simulink library "HybridFEMLibrary"  (Simulink 7.0)
values from neighbouring files (symbols this model uses):
  SampleRate = Integrator.Timestep    [HybridFEMSetupExample.m]
undefined symbols (not defined in the file or in its folder): Elements
libraries: simulink x2
settings Model: Creator=Tommy  LastModifiedBy=Tommy

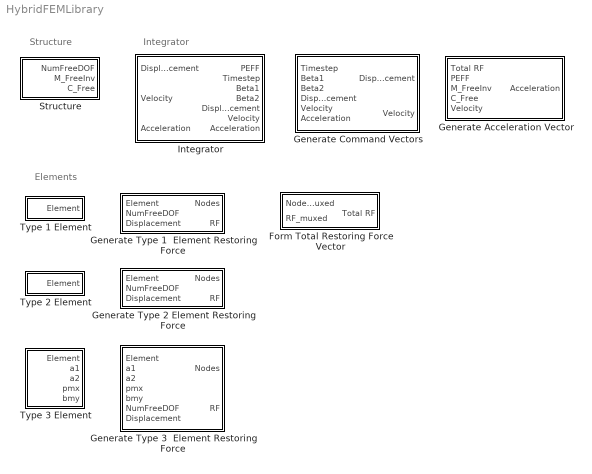
== system HybridFEMLibrary ==
  note: Elements
  note: Structure
  note: Integrator
  Form Total Restoring Force Vector : Subsystem
      mask Type: Form Restoring Force Vector
      mask Description:
      | Takes the restoring force vectors from each Element and combines them to form a total restoring force vector.
      | 
      | Connect the "Nodes_muxed" signal to the output of a Mux block which takes in all the Element "Nodes" outputs in order of ID.
      | 
      | Connect the "RF_muxed" signal to the output of a Mux block which takes in all the Element "RF" outputs in order of ID.
  Generate Acceleration Vector : Subsystem
      mask Type: Generate Acceleration Vector
      mask Description:
      | Takes the total restoring force vector and Integration parameters and generates the next step acceleration vector.
      | 
      | Connect the "Total RF" input to the output of the "Form Total Restoring Force Vector" block.
      | 
      | Connect the "PEFF", "M_Free_Inv" (MassMatrixFreeInv) and "C_Free" (DampingMatrixFree) to the "Structure" block.
      | 
      | Connect the "Velocity" input to the output of the "Generate Command Vectors" block
  Generate Command Vectors : Subsystem
      mask Type: Generate Command Vectors
      mask Description:
      | Generates the Displacement and Velocity vectors using the CR Algorithm.
      | 
      | Connect all inputs to the outputs of the "Integrator" block.
  Generate Type 1  Element Restoring Force : Subsystem
      mask Type: Generate Type 1 Element Restoring Force
      mask Description:
      | Generates the Restoring Force vector for a Type 1 Element
      | 
      | Connect the "Element" input to a "Type 1 Element" block.
      | 
      | Connect the "NumFreeDOF" input to the output of a "Structure" block.
      | 
      | Connect the "Displacement" input to the output of the "Generate Command Vectors" block.
  Generate Type 2 Element Restoring Force : Subsystem
      mask Type: Generate Type 2 Element Restoring Force
      mask Description:
      | Generates the Restoring Force vector for a Type 2 Element
      | 
      | Connect the "Element" input to a "Type 2 Element" block.
      | 
      | Connect the "NumFreeDOF" input to the output of a "Structure" block.
      | 
      | Connect the "Displacement" input to the output of the "Generate Command Vectors" block.
  Generate Type 3  Element Restoring Force : Subsystem
      mask Type: Generate Type 3 Element Restoring Force
      mask Description:
      | Generates the Restoring Force vector for a Type 3 Element
      | 
      | Connect the "Element" input to a "Type 3 Element" block.
      | 
      | Connect the "a1", "a2", "pmx" and "bmy" inputs to the outputs of the "Type 3 Element" block.
      | 
      | Connect the "NumFreeDOF" input to the output of a "Structure" block.
      | 
      | Connect the "Displacement" input to the output of the "Generate Command Vectors" block.
  Integrator : Subsystem
      mask Type: Integrator
      mask Description:
      | The Integrator structure is pulled from the MATLAB workspace after running the initialization script.
      | 
      | Connect the Displacement and Velocity inputs to the outputs of the "Generate Command Vectors" block.
      | 
      | Connect the Acceleration input to the output of the "Generate Acceleration Vector" block
  Structure : Subsystem
      mask Type: Structure Data Source
      mask Description: The Structure data is pulled from the MATLAB workspace after running the initialization file
  "Type 1 Element " : Subsystem  mask(Element Type 1){id=1}
      mask prompts: id "Element ID:"
      mask help: Enter the ID for this element corresponding with the input configuration file
  Type 2 Element : Subsystem  mask(Element Type 2){id=7}
      mask prompts: id "Element ID:"
      mask help: Enter the ID for this element corresponding with the input configuration file
  "Type 3 Element " : Subsystem  mask(Element Type 3){id=0}
      mask prompts: id "Element ID:"
      mask help: Enter the ID for this element corresponding with the input configuration file

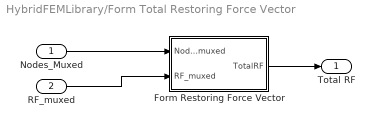
== system HybridFEMLibrary/Form Total Restoring Force Vector ==
  Nodes_Muxed : Inport  OutDataType=sfix(16)  OutScaling=2^0
  RF_muxed : Inport  Port=2  OutDataType=sfix(16)  OutScaling=2^0
  Form Restoring Force Vector : Stateflow chart
  Total RF : Outport  OutDataType=sfix(16)  OutScaling=2^0
  wires:
  Nodes_Muxed/1 -> Form Restoring Force Vector/1(Nodes_muxed)
  Form Restoring Force Vector/1(TotalRF) -> Total RF/1
  RF_muxed/1 -> Form Restoring Force Vector/2(RF_muxed)

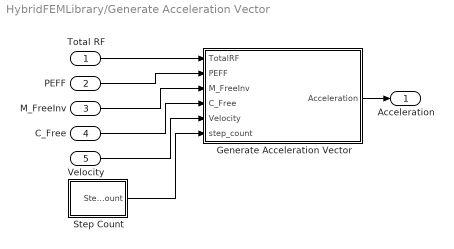
== system HybridFEMLibrary/Generate Acceleration Vector ==
  Total RF : Inport  OutDataType=sfix(16)  OutScaling=2^0
  PEFF : Inport  Port=2  OutDataType=sfix(16)  OutScaling=2^0
  M_FreeInv : Inport  Port=3  OutDataType=sfix(16)  OutScaling=2^0
  C_Free : Inport  Port=4  OutDataType=sfix(16)  OutScaling=2^0
  Velocity : Inport  Port=5  OutDataType=sfix(16)  OutScaling=2^0
  Generate Acceleration Vector : Stateflow chart
  Step Count : Subsystem
      mask Type: Step count
      mask Description: Generates the step count
  Acceleration : Outport  OutDataType=sfix(16)  OutScaling=2^0
  wires:
  Velocity/1 -> Generate Acceleration Vector/5(Velocity)
  C_Free/1 -> Generate Acceleration Vector/4(C_Free)
  M_FreeInv/1 -> Generate Acceleration Vector/3(M_FreeInv)
  PEFF/1 -> Generate Acceleration Vector/2(PEFF)
  Generate Acceleration Vector/1(Acceleration) -> Acceleration/1
  Total RF/1 -> Generate Acceleration Vector/1(TotalRF)
  Step Count/1(Step Count) -> Generate Acceleration Vector/6(step_count)

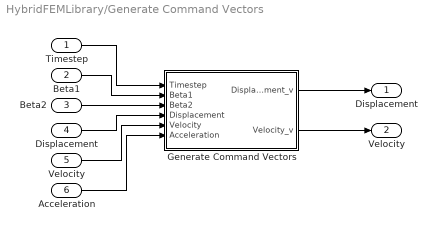
== system HybridFEMLibrary/Generate Command Vectors ==
  Timestep : Inport  OutDataType=sfix(16)  OutScaling=2^0
  Beta1 : Inport  Port=2  OutDataType=sfix(16)  OutScaling=2^0
  Beta2 : Inport  Port=3  OutDataType=sfix(16)  OutScaling=2^0
  "Displacement " : Inport  Port=4  OutDataType=sfix(16)  OutScaling=2^0
  "Velocity " : Inport  Port=5  OutDataType=sfix(16)  OutScaling=2^0
  Acceleration : Inport  Port=6  OutDataType=sfix(16)  OutScaling=2^0
  Generate Command Vectors : Stateflow chart
  Displacement : Outport  OutDataType=sfix(16)  OutScaling=2^0
  Velocity : Outport  Port=2  OutDataType=sfix(16)  OutScaling=2^0
  wires:
  Acceleration/1 -> Generate Command Vectors/6(Acceleration)
  "Velocity "/1 -> Generate Command Vectors/5(Velocity)
  "Displacement "/1 -> Generate Command Vectors/4(Displacement)
  Beta2/1 -> Generate Command Vectors/3(Beta2)
  Beta1/1 -> Generate Command Vectors/2(Beta1)
  Timestep/1 -> Generate Command Vectors/1(Timestep)
  Generate Command Vectors/2(Velocity_v) -> Velocity/1
  Generate Command Vectors/1(Displacement_v) -> Displacement/1

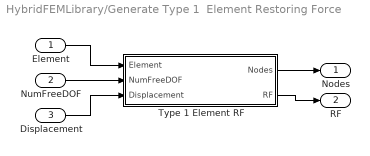
== system HybridFEMLibrary/Generate Type 1  Element Restoring Force ==
  Element : Inport  OutDataType=sfix(16)  OutScaling=2^0
  NumFreeDOF : Inport  Port=2  OutDataType=sfix(16)  OutScaling=2^0
  Displacement : Inport  Port=3  OutDataType=sfix(16)  OutScaling=2^0
  Type 1 Element RF : Stateflow chart
  Nodes : Outport  OutDataType=sfix(16)  OutScaling=2^0
  RF : Outport  Port=2  OutDataType=sfix(16)  OutScaling=2^0
  wires:
  Displacement/1 -> Type 1 Element RF/3(Displacement)
  NumFreeDOF/1 -> Type 1 Element RF/2(NumFreeDOF)
  Element/1 -> Type 1 Element RF/1(Element)
  Type 1 Element RF/2(RF) -> RF/1
  Type 1 Element RF/1(Nodes) -> Nodes/1

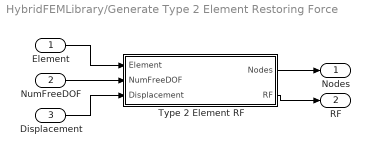
== system HybridFEMLibrary/Generate Type 2 Element Restoring Force ==
  Element : Inport  OutDataType=sfix(16)  OutScaling=2^0
  NumFreeDOF : Inport  Port=2  OutDataType=sfix(16)  OutScaling=2^0
  Displacement : Inport  Port=3  OutDataType=sfix(16)  OutScaling=2^0
  Type 2 Element RF : Stateflow chart
  Nodes : Outport  OutDataType=sfix(16)  OutScaling=2^0
  RF : Outport  Port=2  OutDataType=sfix(16)  OutScaling=2^0
  wires:
  Type 2 Element RF/1(Nodes) -> Nodes/1
  Type 2 Element RF/2(RF) -> RF/1
  Element/1 -> Type 2 Element RF/1(Element)
  NumFreeDOF/1 -> Type 2 Element RF/2(NumFreeDOF)
  Displacement/1 -> Type 2 Element RF/3(Displacement)

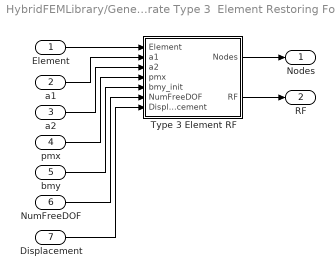
== system HybridFEMLibrary/Generate Type 3  Element Restoring Force ==
  Element : Inport  OutDataType=sfix(16)  OutScaling=2^0
  a1 : Inport  Port=2  OutDataType=sfix(16)  OutScaling=2^0
  a2 : Inport  Port=3  OutDataType=sfix(16)  OutScaling=2^0
  pmx : Inport  Port=4  OutDataType=sfix(16)  OutScaling=2^0
  bmy : Inport  Port=5  OutDataType=sfix(16)  OutScaling=2^0
  NumFreeDOF : Inport  Port=6  OutDataType=sfix(16)  OutScaling=2^0
  Displacement : Inport  Port=7  OutDataType=sfix(16)  OutScaling=2^0
  Type 3 Element RF : Stateflow chart
  Nodes : Outport  OutDataType=sfix(16)  OutScaling=2^0
  RF : Outport  Port=2  OutDataType=sfix(16)  OutScaling=2^0
  wires:
  Displacement/1 -> Type 3 Element RF/7(Displacement)
  NumFreeDOF/1 -> Type 3 Element RF/6(NumFreeDOF)
  bmy/1 -> Type 3 Element RF/5(bmy_init)
  pmx/1 -> Type 3 Element RF/4(pmx)
  a2/1 -> Type 3 Element RF/3(a2)
  a1/1 -> Type 3 Element RF/2(a1)
  Element/1 -> Type 3 Element RF/1(Element)
  Type 3 Element RF/2(RF) -> RF/1
  Type 3 Element RF/1(Nodes) -> Nodes/1

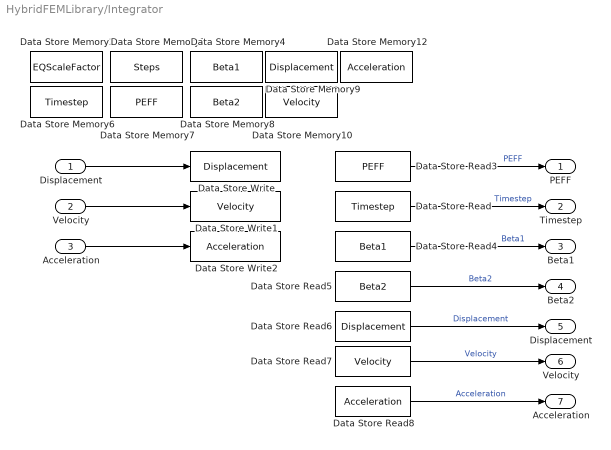
== system HybridFEMLibrary/Integrator ==
  "Displacement " : Inport  OutDataType=sfix(16)  OutScaling=2^0
  "Velocity " : Inport  Port=2  OutDataType=sfix(16)  OutScaling=2^0
  "Acceleration " : Inport  Port=3  OutDataType=sfix(16)  OutScaling=2^0
  Data Store Memory10 : DataStoreMemory  DataStoreName=Velocity  InitialValue=Integrator.Velocity  OutDataType=sfix(16)  OutScaling=2^0
  Data Store Memory12 : DataStoreMemory  DataStoreName=Acceleration  InitialValue=Integrator.Acceleration  OutDataType=sfix(16)  OutScaling=2^0
  Data Store Memory2 : DataStoreMemory  DataStoreName=EQScaleFactor  InitialValue=Integrator.EQScaleFactor  OutDataType=sfix(16)  OutScaling=2^0
  Data Store Memory3 : DataStoreMemory  DataStoreName=Steps  InitialValue=Integrator.Steps  OutDataType=sfix(16)  OutScaling=2^0
  Data Store Memory4 : DataStoreMemory  DataStoreName=Beta1  InitialValue=Integrator.Beta1  OutDataType=sfix(16)  OutScaling=2^0
  Data Store Memory6 : DataStoreMemory  DataStoreName=Timestep  InitialValue=Integrator.Timestep  OutDataType=sfix(16)  OutScaling=2^0
  Data Store Memory7 : DataStoreMemory  DataStoreName=PEFF  InitialValue=Integrator.PEFF  OutDataType=sfix(16)  OutScaling=2^0
  Data Store Memory8 : DataStoreMemory  DataStoreName=Beta2  InitialValue=Integrator.Beta2  OutDataType=sfix(16)  OutScaling=2^0
  Data Store Memory9 : DataStoreMemory  DataStoreName=Displacement  InitialValue=Integrator.Displacement  OutDataType=sfix(16)  OutScaling=2^0
  Data Store Read : DataStoreRead  DataStoreName=Timestep  SampleTime=SampleRate
  Data Store Read3 : DataStoreRead  DataStoreName=PEFF  SampleTime=SampleRate
  Data Store Read4 : DataStoreRead  DataStoreName=Beta1  SampleTime=SampleRate
  Data Store Read5 : DataStoreRead  DataStoreName=Beta2  SampleTime=SampleRate
  Data Store Read6 : DataStoreRead  DataStoreName=Displacement  SampleTime=SampleRate
  Data Store Read7 : DataStoreRead  DataStoreName=Velocity  SampleTime=SampleRate
  Data Store Read8 : DataStoreRead  DataStoreName=Acceleration  SampleTime=SampleRate
  Data Store Write : DataStoreWrite  DataStoreName=Displacement  SampleTime=SampleRate
  Data Store Write1 : DataStoreWrite  DataStoreName=Velocity  SampleTime=SampleRate
  Data Store Write2 : DataStoreWrite  DataStoreName=Acceleration  SampleTime=SampleRate
  PEFF : Outport  OutDataType=sfix(16)  OutScaling=2^0
  Timestep : Outport  Port=2  OutDataType=sfix(16)  OutScaling=2^0
  Beta1 : Outport  Port=3  OutDataType=sfix(16)  OutScaling=2^0
  Beta2 : Outport  Port=4  OutDataType=sfix(16)  OutScaling=2^0
  Displacement : Outport  Port=5  OutDataType=sfix(16)  OutScaling=2^0
  Velocity : Outport  Port=6  OutDataType=sfix(16)  OutScaling=2^0
  Acceleration : Outport  Port=7  OutDataType=sfix(16)  OutScaling=2^0
  wires:
  Data Store Read8/1 -> Acceleration/1  "Acceleration"
  Data Store Read7/1 -> Velocity/1  "Velocity"
  Data Store Read6/1 -> Displacement/1  "Displacement"
  Data Store Read5/1 -> Beta2/1  "Beta2"
  Data Store Read4/1 -> Beta1/1  "Beta1"
  Data Store Read3/1 -> PEFF/1  "PEFF"
  "Displacement "/1 -> Data Store Write/1
  "Velocity "/1 -> Data Store Write1/1
  "Acceleration "/1 -> Data Store Write2/1
  Data Store Read/1 -> Timestep/1  "Timestep"

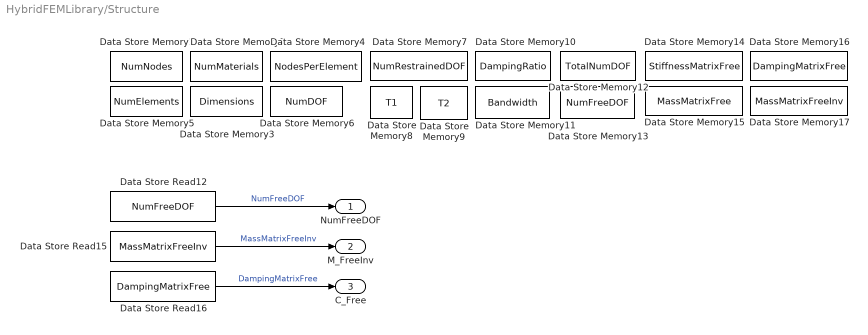
== system HybridFEMLibrary/Structure ==
  Data Store Memory1 : DataStoreMemory  DataStoreName=NumNodes  InitialValue=Structure.NumNodes  OutDataType=sfix(16)  OutScaling=2^0
  Data Store Memory10 : DataStoreMemory  DataStoreName=DampingRatio  InitialValue=Structure.DampingRatio  OutDataType=sfix(16)  OutScaling=2^0
  Data Store Memory11 : DataStoreMemory  DataStoreName=Bandwidth  InitialValue=Structure.Bandwidth  OutDataType=sfix(16)  OutScaling=2^0
  Data Store Memory12 : DataStoreMemory  DataStoreName=TotalNumDOF  InitialValue=Structure.TotalNumDOF  OutDataType=sfix(16)  OutScaling=2^0
  Data Store Memory13 : DataStoreMemory  DataStoreName=NumFreeDOF  InitialValue=Structure.NumFreeDOF  OutDataType=sfix(16)  OutScaling=2^0
  Data Store Memory14 : DataStoreMemory  DataStoreName=StiffnessMatrixFree  InitialValue=Structure.StiffnessMatrixFree  OutDataType=sfix(16)  OutScaling=2^0
  Data Store Memory15 : DataStoreMemory  DataStoreName=MassMatrixFree  InitialValue=Structure.MassMatrixFree  OutDataType=sfix(16)  OutScaling=2^0
  Data Store Memory16 : DataStoreMemory  DataStoreName=DampingMatrixFree  InitialValue=Structure.DampingMatrixFree  OutDataType=sfix(16)  OutScaling=2^0
  Data Store Memory17 : DataStoreMemory  DataStoreName=MassMatrixFreeInv  InitialValue=Structure.MassMatrixFreeInv  OutDataType=sfix(16)  OutScaling=2^0
  Data Store Memory2 : DataStoreMemory  DataStoreName=NumMaterials  InitialValue=Structure.NumMaterials  OutDataType=sfix(16)  OutScaling=2^0
  Data Store Memory3 : DataStoreMemory  DataStoreName=Dimensions  InitialValue=Structure.Dimensions  OutDataType=sfix(16)  OutScaling=2^0
  Data Store Memory4 : DataStoreMemory  DataStoreName=NodesPerElement  InitialValue=Structure.NodesPerElement  OutDataType=sfix(16)  OutScaling=2^0
  Data Store Memory5 : DataStoreMemory  DataStoreName=NumElements  InitialValue=Structure.NumElements  OutDataType=sfix(16)  OutScaling=2^0
  Data Store Memory6 : DataStoreMemory  DataStoreName=NumDOF  InitialValue=Structure.NumDOF  OutDataType=sfix(16)  OutScaling=2^0
  Data Store Memory7 : DataStoreMemory  DataStoreName=NumRestrainedDOF  InitialValue=Structure.NumRestrainedDOF  OutDataType=sfix(16)  OutScaling=2^0
  Data Store Memory8 : DataStoreMemory  DataStoreName=T1  InitialValue=Structure.T1  OutDataType=sfix(16)  OutScaling=2^0
  Data Store Memory9 : DataStoreMemory  DataStoreName=T2  InitialValue=Structure.T2  OutDataType=sfix(16)  OutScaling=2^0
  Data Store Read12 : DataStoreRead  DataStoreName=NumFreeDOF  SampleTime=SampleRate
  Data Store Read15 : DataStoreRead  DataStoreName=MassMatrixFreeInv  SampleTime=SampleRate
  Data Store Read16 : DataStoreRead  DataStoreName=DampingMatrixFree  SampleTime=SampleRate
  NumFreeDOF : Outport  OutDataType=sfix(16)  OutScaling=2^0
  M_FreeInv : Outport  Port=2  OutDataType=sfix(16)  OutScaling=2^0
  C_Free : Outport  Port=3  OutDataType=sfix(16)  OutScaling=2^0
  wires:
  Data Store Read16/1 -> C_Free/1  "DampingMatrixFree"
  Data Store Read15/1 -> M_FreeInv/1  "MassMatrixFreeInv"
  Data Store Read12/1 -> NumFreeDOF/1  "NumFreeDOF"

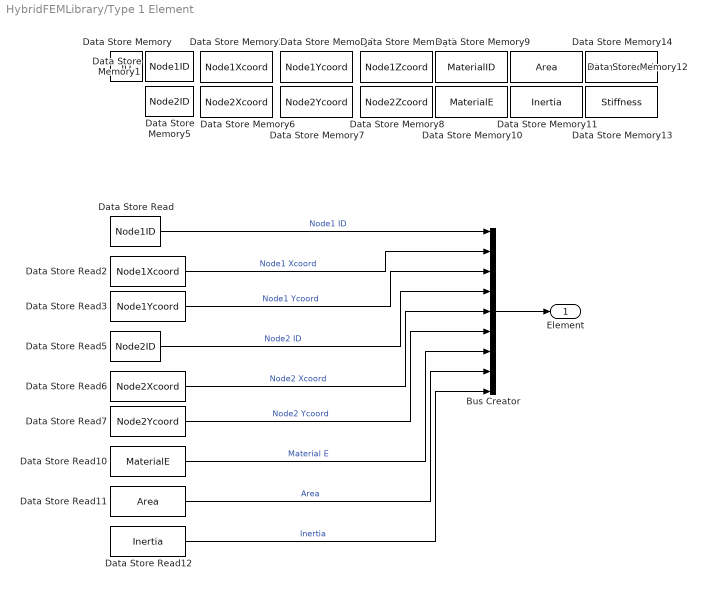
== system HybridFEMLibrary/Type 1 Element  ==
  Bus Creator : BusCreator  Inputs=9
  Data Store Memory : DataStoreMemory  DataStoreName=ID  InitialValue=Elements(id).ID  OutDataType=sfix(16)  OutScaling=2^0
  Data Store Memory1 : DataStoreMemory  DataStoreName=Node1ID  InitialValue=Elements(id).Nodes(1).ID  OutDataType=sfix(16)  OutScaling=2^0
  Data Store Memory10 : DataStoreMemory  DataStoreName=MaterialE  InitialValue=Elements(id).Material(1).E  OutDataType=sfix(16)  OutScaling=2^0
  Data Store Memory11 : DataStoreMemory  DataStoreName=Inertia  InitialValue=Elements(id).Inertia  OutDataType=sfix(16)  OutScaling=2^0
  Data Store Memory12 : DataStoreMemory  DataStoreName=Area  InitialValue=Elements(id).Area  OutDataType=sfix(16)  OutScaling=2^0
  Data Store Memory13 : DataStoreMemory  DataStoreName=Stiffness  InitialValue=Elements(id).Stiffness  OutDataType=sfix(16)  OutScaling=2^0
  Data Store Memory14 : DataStoreMemory  DataStoreName=ElemDistLoad  InitialValue=Elements(id).ElemDistLoad  OutDataType=sfix(16)  OutScaling=2^0
  Data Store Memory2 : DataStoreMemory  DataStoreName=Node1Xcoord  InitialValue=Elements(id).Nodes(1).Xcoord  OutDataType=sfix(16)  OutScaling=2^0
  Data Store Memory3 : DataStoreMemory  DataStoreName=Node1Ycoord  InitialValue=Elements(id).Nodes(1).Ycoord  OutDataType=sfix(16)  OutScaling=2^0
  Data Store Memory4 : DataStoreMemory  DataStoreName=Node1Zcoord  InitialValue=Elements(id).Nodes(1).Zcoord  OutDataType=sfix(16)  OutScaling=2^0
  Data Store Memory5 : DataStoreMemory  DataStoreName=Node2ID  InitialValue=Elements(id).Nodes(2).ID  OutDataType=sfix(16)  OutScaling=2^0
  Data Store Memory6 : DataStoreMemory  DataStoreName=Node2Xcoord  InitialValue=Elements(id).Nodes(2).Xcoord  OutDataType=sfix(16)  OutScaling=2^0
  Data Store Memory7 : DataStoreMemory  DataStoreName=Node2Ycoord  InitialValue=Elements(id).Nodes(2).Ycoord  OutDataType=sfix(16)  OutScaling=2^0
  Data Store Memory8 : DataStoreMemory  DataStoreName=Node2Zcoord  InitialValue=Elements(id).Nodes(2).Zcoord  OutDataType=sfix(16)  OutScaling=2^0
  Data Store Memory9 : DataStoreMemory  DataStoreName=MaterialID  InitialValue=Elements(id).Material(1).ID  OutDataType=sfix(16)  OutScaling=2^0
  Data Store Read : DataStoreRead  DataStoreName=Node1ID  SampleTime=SampleRate
  Data Store Read10 : DataStoreRead  DataStoreName=MaterialE  SampleTime=SampleRate
  Data Store Read11 : DataStoreRead  DataStoreName=Area  SampleTime=SampleRate
  Data Store Read12 : DataStoreRead  DataStoreName=Inertia  SampleTime=SampleRate
  Data Store Read2 : DataStoreRead  DataStoreName=Node1Xcoord  SampleTime=SampleRate
  Data Store Read3 : DataStoreRead  DataStoreName=Node1Ycoord  SampleTime=SampleRate
  Data Store Read5 : DataStoreRead  DataStoreName=Node2ID  SampleTime=SampleRate
  Data Store Read6 : DataStoreRead  DataStoreName=Node2Xcoord  SampleTime=SampleRate
  Data Store Read7 : DataStoreRead  DataStoreName=Node2Ycoord  SampleTime=SampleRate
  Element : Outport  OutDataType=sfix(16)  OutScaling=2^0
  wires:
  Data Store Read12/1 -> Bus Creator/9  "Inertia"
  Data Store Read11/1 -> Bus Creator/8  "Area"
  Data Store Read10/1 -> Bus Creator/7  "Material E"
  Data Store Read7/1 -> Bus Creator/6  "Node2 Ycoord"
  Data Store Read6/1 -> Bus Creator/5  "Node2 Xcoord"
  Data Store Read5/1 -> Bus Creator/4  "Node2 ID"
  Data Store Read3/1 -> Bus Creator/3  "Node1 Ycoord"
  Data Store Read2/1 -> Bus Creator/2  "Node1 Xcoord"
  Data Store Read/1 -> Bus Creator/1  "Node1 ID"
  Bus Creator/1 -> Element/1

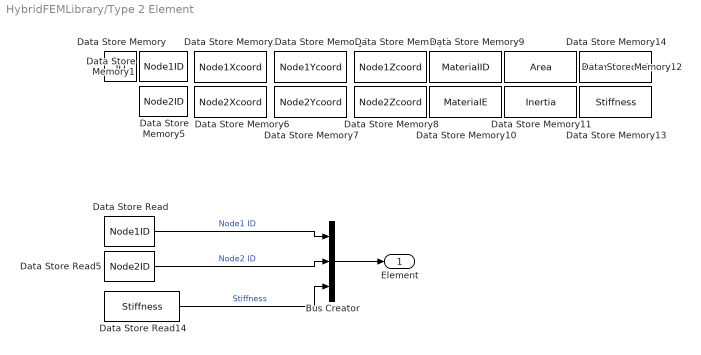
== system HybridFEMLibrary/Type 2 Element ==
  Bus Creator : BusCreator  Inputs=3
  Data Store Memory : DataStoreMemory  DataStoreName=ID  InitialValue=Elements(id).ID  OutDataType=sfix(16)  OutScaling=2^0
  Data Store Memory1 : DataStoreMemory  DataStoreName=Node1ID  InitialValue=Elements(id).Nodes(1).ID  OutDataType=sfix(16)  OutScaling=2^0
  Data Store Memory10 : DataStoreMemory  DataStoreName=MaterialE  InitialValue=Elements(id).Material(1).E  OutDataType=sfix(16)  OutScaling=2^0
  Data Store Memory11 : DataStoreMemory  DataStoreName=Inertia  InitialValue=Elements(id).Inertia  OutDataType=sfix(16)  OutScaling=2^0
  Data Store Memory12 : DataStoreMemory  DataStoreName=Area  InitialValue=Elements(id).Area  OutDataType=sfix(16)  OutScaling=2^0
  Data Store Memory13 : DataStoreMemory  DataStoreName=Stiffness  InitialValue=Elements(id).Stiffness  OutDataType=sfix(16)  OutScaling=2^0
  Data Store Memory14 : DataStoreMemory  DataStoreName=ElemDistLoad  InitialValue=Elements(id).ElemDistLoad  OutDataType=sfix(16)  OutScaling=2^0
  Data Store Memory2 : DataStoreMemory  DataStoreName=Node1Xcoord  InitialValue=Elements(id).Nodes(1).Xcoord  OutDataType=sfix(16)  OutScaling=2^0
  Data Store Memory3 : DataStoreMemory  DataStoreName=Node1Ycoord  InitialValue=Elements(id).Nodes(1).Ycoord  OutDataType=sfix(16)  OutScaling=2^0
  Data Store Memory4 : DataStoreMemory  DataStoreName=Node1Zcoord  InitialValue=Elements(id).Nodes(1).Zcoord  OutDataType=sfix(16)  OutScaling=2^0
  Data Store Memory5 : DataStoreMemory  DataStoreName=Node2ID  InitialValue=Elements(id).Nodes(2).ID  OutDataType=sfix(16)  OutScaling=2^0
  Data Store Memory6 : DataStoreMemory  DataStoreName=Node2Xcoord  InitialValue=Elements(id).Nodes(2).Xcoord  OutDataType=sfix(16)  OutScaling=2^0
  Data Store Memory7 : DataStoreMemory  DataStoreName=Node2Ycoord  InitialValue=Elements(id).Nodes(2).Ycoord  OutDataType=sfix(16)  OutScaling=2^0
  Data Store Memory8 : DataStoreMemory  DataStoreName=Node2Zcoord  InitialValue=Elements(id).Nodes(2).Zcoord  OutDataType=sfix(16)  OutScaling=2^0
  Data Store Memory9 : DataStoreMemory  DataStoreName=MaterialID  InitialValue=Elements(id).Material(1).ID  OutDataType=sfix(16)  OutScaling=2^0
  Data Store Read : DataStoreRead  DataStoreName=Node1ID  SampleTime=SampleRate
  Data Store Read14 : DataStoreRead  DataStoreName=Stiffness  SampleTime=SampleRate
  Data Store Read5 : DataStoreRead  DataStoreName=Node2ID  SampleTime=SampleRate
  Element : Outport  OutDataType=sfix(16)  OutScaling=2^0
  wires:
  Bus Creator/1 -> Element/1
  Data Store Read/1 -> Bus Creator/1  "Node1 ID"
  Data Store Read5/1 -> Bus Creator/2  "Node2 ID"
  Data Store Read14/1 -> Bus Creator/3  "Stiffness"

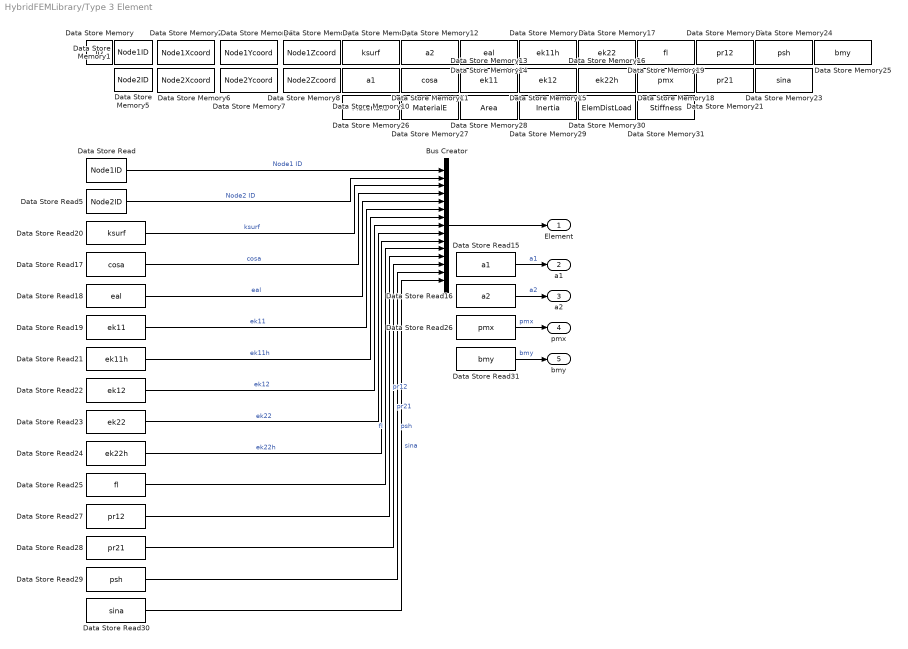
== system HybridFEMLibrary/Type 3 Element  ==
  Bus Creator : BusCreator  Inputs=15
  Data Store Memory : DataStoreMemory  DataStoreName=ID  InitialValue=Elements(id).ID  OutDataType=sfix(16)  OutScaling=2^0
  Data Store Memory1 : DataStoreMemory  DataStoreName=Node1ID  InitialValue=Elements(id).Nodes(1).ID  OutDataType=sfix(16)  OutScaling=2^0
  Data Store Memory10 : DataStoreMemory  DataStoreName=a1  InitialValue=Elements(id).a1  OutDataType=sfix(16)  OutScaling=2^0
  Data Store Memory11 : DataStoreMemory  DataStoreName=cosa  InitialValue=Elements(id).cosa  OutDataType=sfix(16)  OutScaling=2^0
  Data Store Memory12 : DataStoreMemory  DataStoreName=a2  InitialValue=Elements(id).a2  OutDataType=sfix(16)  OutScaling=2^0
  Data Store Memory13 : DataStoreMemory  DataStoreName=ek11  InitialValue=Elements(id).ek11  OutDataType=sfix(16)  OutScaling=2^0
  Data Store Memory14 : DataStoreMemory  DataStoreName=eal  InitialValue=Elements(id).eal  OutDataType=sfix(16)  OutScaling=2^0
  Data Store Memory15 : DataStoreMemory  DataStoreName=ek12  InitialValue=Elements(id).ek12  OutDataType=sfix(16)  OutScaling=2^0
  Data Store Memory16 : DataStoreMemory  DataStoreName=ek22h  InitialValue=Elements(id).ek22h  OutDataType=sfix(16)  OutScaling=2^0
  Data Store Memory17 : DataStoreMemory  DataStoreName=ek22  InitialValue=Elements(id).ek22  OutDataType=sfix(16)  OutScaling=2^0
  Data Store Memory18 : DataStoreMemory  DataStoreName=pmx  InitialValue=Elements(id).pmx  OutDataType=sfix(16)  OutScaling=2^0
  Data Store Memory19 : DataStoreMemory  DataStoreName=fl  InitialValue=Elements(id).fl  OutDataType=sfix(16)  OutScaling=2^0
  Data Store Memory2 : DataStoreMemory  DataStoreName=Node1Xcoord  InitialValue=Elements(id).Nodes(1).Xcoord  OutDataType=sfix(16)  OutScaling=2^0
  Data Store Memory20 : DataStoreMemory  DataStoreName=ek11h  InitialValue=Elements(id).ek11h  OutDataType=sfix(16)  OutScaling=2^0
  Data Store Memory21 : DataStoreMemory  DataStoreName=pr21  InitialValue=Elements(id).pr21  OutDataType=sfix(16)  OutScaling=2^0
  Data Store Memory22 : DataStoreMemory  DataStoreName=pr12  InitialValue=Elements(id).pr12  OutDataType=sfix(16)  OutScaling=2^0
  Data Store Memory23 : DataStoreMemory  DataStoreName=sina  InitialValue=Elements(id).sina  OutDataType=sfix(16)  OutScaling=2^0
  Data Store Memory24 : DataStoreMemory  DataStoreName=psh  InitialValue=Elements(id).psh  OutDataType=sfix(16)  OutScaling=2^0
  Data Store Memory25 : DataStoreMemory  DataStoreName=bmy  InitialValue=Elements(id).bmy  OutDataType=sfix(16)  OutScaling=2^0
  Data Store Memory26 : DataStoreMemory  DataStoreName=MaterialID  InitialValue=Elements(id).Material.ID  OutDataType=sfix(16)  OutScaling=2^0
  Data Store Memory27 : DataStoreMemory  DataStoreName=MaterialE  InitialValue=Elements(id).Material.E  OutDataType=sfix(16)  OutScaling=2^0
  Data Store Memory28 : DataStoreMemory  DataStoreName=Area  InitialValue=Elements(id).Area  OutDataType=sfix(16)  OutScaling=2^0
  Data Store Memory29 : DataStoreMemory  DataStoreName=Inertia  InitialValue=Elements(id).Inertia  OutDataType=sfix(16)  OutScaling=2^0
  Data Store Memory3 : DataStoreMemory  DataStoreName=Node1Ycoord  InitialValue=Elements(id).Nodes(1).Ycoord  OutDataType=sfix(16)  OutScaling=2^0
  Data Store Memory30 : DataStoreMemory  DataStoreName=ElemDistLoad  InitialValue=Elements(id).ElemDistLoad  OutDataType=sfix(16)  OutScaling=2^0
  Data Store Memory31 : DataStoreMemory  DataStoreName=Stiffness  InitialValue=Elements(id).Stiffness  OutDataType=sfix(16)  OutScaling=2^0
  Data Store Memory4 : DataStoreMemory  DataStoreName=Node1Zcoord  InitialValue=Elements(id).Nodes(1).Zcoord  OutDataType=sfix(16)  OutScaling=2^0
  Data Store Memory5 : DataStoreMemory  DataStoreName=Node2ID  InitialValue=Elements(id).Nodes(2).ID  OutDataType=sfix(16)  OutScaling=2^0
  Data Store Memory6 : DataStoreMemory  DataStoreName=Node2Xcoord  InitialValue=Elements(id).Nodes(2).Xcoord  OutDataType=sfix(16)  OutScaling=2^0
  Data Store Memory7 : DataStoreMemory  DataStoreName=Node2Ycoord  InitialValue=Elements(id).Nodes(2).Ycoord  OutDataType=sfix(16)  OutScaling=2^0
  Data Store Memory8 : DataStoreMemory  DataStoreName=Node2Zcoord  InitialValue=Elements(id).Nodes(2).Zcoord  OutDataType=sfix(16)  OutScaling=2^0
  Data Store Memory9 : DataStoreMemory  DataStoreName=ksurf  InitialValue=Elements(id).ksurf  OutDataType=sfix(16)  OutScaling=2^0
  Data Store Read : DataStoreRead  DataStoreName=Node1ID  SampleTime=SampleRate
  Data Store Read15 : DataStoreRead  DataStoreName=a1  SampleTime=SampleRate
  Data Store Read16 : DataStoreRead  DataStoreName=a2  SampleTime=SampleRate
  Data Store Read17 : DataStoreRead  DataStoreName=cosa  SampleTime=SampleRate
  Data Store Read18 : DataStoreRead  DataStoreName=eal  SampleTime=SampleRate
  Data Store Read19 : DataStoreRead  DataStoreName=ek11  SampleTime=SampleRate
  Data Store Read20 : DataStoreRead  DataStoreName=ksurf  SampleTime=SampleRate
  Data Store Read21 : DataStoreRead  DataStoreName=ek11h  SampleTime=SampleRate
  Data Store Read22 : DataStoreRead  DataStoreName=ek12  SampleTime=SampleRate
  Data Store Read23 : DataStoreRead  DataStoreName=ek22  SampleTime=SampleRate
  Data Store Read24 : DataStoreRead  DataStoreName=ek22h  SampleTime=SampleRate
  Data Store Read25 : DataStoreRead  DataStoreName=fl  SampleTime=SampleRate
  Data Store Read26 : DataStoreRead  DataStoreName=pmx  SampleTime=SampleRate
  Data Store Read27 : DataStoreRead  DataStoreName=pr12  SampleTime=SampleRate
  Data Store Read28 : DataStoreRead  DataStoreName=pr21  SampleTime=SampleRate
  Data Store Read29 : DataStoreRead  DataStoreName=psh  SampleTime=SampleRate
  Data Store Read30 : DataStoreRead  DataStoreName=sina  SampleTime=SampleRate
  Data Store Read31 : DataStoreRead  DataStoreName=bmy  SampleTime=SampleRate
  Data Store Read5 : DataStoreRead  DataStoreName=Node2ID  SampleTime=SampleRate
  Element : Outport  OutDataType=sfix(16)  OutScaling=2^0
  a1 : Outport  Port=2  OutDataType=sfix(16)  OutScaling=2^0
  a2 : Outport  Port=3  OutDataType=sfix(16)  OutScaling=2^0
  pmx : Outport  Port=4  OutDataType=sfix(16)  OutScaling=2^0
  bmy : Outport  Port=5  OutDataType=sfix(16)  OutScaling=2^0
  wires:
  Data Store Read31/1 -> bmy/1  "bmy"
  Data Store Read26/1 -> pmx/1  "pmx"
  Data Store Read16/1 -> a2/1  "a2"
  Data Store Read15/1 -> a1/1  "a1"
  Data Store Read30/1 -> Bus Creator/15  "sina"
  Data Store Read29/1 -> Bus Creator/14  "psh"
  Data Store Read28/1 -> Bus Creator/13  "pr21"
  Data Store Read27/1 -> Bus Creator/12  "pr12"
  Data Store Read25/1 -> Bus Creator/11  "fl"
  Data Store Read24/1 -> Bus Creator/10  "ek22h"
  Data Store Read23/1 -> Bus Creator/9  "ek22"
  Data Store Read22/1 -> Bus Creator/8  "ek12"
  Data Store Read21/1 -> Bus Creator/7  "ek11h"
  Data Store Read19/1 -> Bus Creator/6  "ek11"
  Data Store Read18/1 -> Bus Creator/5  "eal"
  Data Store Read17/1 -> Bus Creator/4  "cosa"
  Data Store Read20/1 -> Bus Creator/3  "ksurf"
  Data Store Read5/1 -> Bus Creator/2  "Node2 ID"
  Data Store Read/1 -> Bus Creator/1  "Node1 ID"
  Bus Creator/1 -> Element/1

== system HybridFEMLibrary/Generate Acceleration Vector/Step Count ==
  Increment Stored Integer : simulink/Additional Math & Discrete/Additional Math: Increment - Decrement/Increment Stored Integer  SystemSampleTime=-1
  step count : simulink/Sources/Counter Free-Running  SystemSampleTime=-1  NumBits=32  tsamp=SampleRate
  Step Count : Outport  OutDataType=sfix(16)  OutScaling=2^0
  wires:
  Increment Stored Integer/1 -> Step Count/1
  step count/1 -> Increment Stored Integer/1

== matlab function Generate Type 3 Element Restoring Force/Type 3 Element RF ==
  data: Nodes output inherited; Element input inherited; a1 input inherited; a2 input inherited; pmx input inherited; bmy_init input inherited; RF output inherited; NumFreeDOF input inherited; Displacement input inherited
% Get Restoring Force Type 3
function [Nodes,RF] = fnc(Element, a1, a2, pmx, bmy_init, NumFreeDOF, Displacement)

persistent initialized;
persistent kody;
persistent bmep;
persistent bmel;
persistent bmtot;
persistent bbmy;
persistent dpr;
persistent bmy;
persistent ftot;
persistent pracn;
persistent pracp;
persistent prtot;
persistent sftot;
persistent Uprev;

%% Input mapping
Node1ID = Element(1);
Node2ID = Element(2);
Nodes = [Node1ID,Node2ID];
ksurf = Element(3);
cosa = Element(4);
eal = Element(5);
ek11 = Element(6);
ek11h = Element(7);
ek12 = Element(8);
ek22 = Element(9);
ek22h = Element(10);
fl = Element(11);
pr12 = Element(12);
pr21 = Element(13);
psh = Element(14);
sina = Element(15);

if isempty(initialized)
    initialized = 1;
    kody = zeros(2,1);
    bmep = zeros(2,1); 
    bmel = zeros(2,1);
    bmtot = zeros(2,1);
    bbmy = 0;
    dpr = zeros(2,1);
    ftot = zeros(2,1);  
    pracn = zeros(2,1); 
    pracp = zeros(2,1);
    prtot = zeros(2,1);
    sftot = zeros(2,1); 
    Uprev = zeros(6,1);
    bmy = bmy_init;
end



%% Get distance between nodes
I1 = Node1ID; %Node1ID;
I2 = Node2ID; %Node2ID;

%% Get the displacement Ue (6x1) vector of the element in global coordinates
Ue = zeros(6,1);
if (I1 * 3) <= NumFreeDOF
    Ue(1, 1) = Displacement(I1 * 3 - 2, 1);
    Ue(2, 1) = Displacement(I1 * 3 - 1, 1);
    Ue(3, 1) = Displacement(I1 * 3, 1);
end
if (I2 * 3) <= NumFreeDOF
    Ue(4, 1) = Displacement(I2 * 3 - 2, 1);
    Ue(5, 1) = Displacement(I2 * 3 - 1, 1);
    Ue(6, 1) = Displacement(I2 * 3, 1);
end

%% Input of Drain State Determination Type 2 Element
ndof=6;  %the element has 6 dofs
ddise=Ue-Uprev;  %the incremental displacement vector ddise of the element in global coordinates 
Uprev=Ue; %update Uprev of element for use in next state determination call
%% calculate element deformation increments
[dvax,dvr] = ELDFO2(ddise,fl,cosa,sina);
%% UPDATE AXIAL FORCES AND AXIAL ENERGY
dfax=eal*dvax;      
ftot(1,1)=ftot(1,1)-dfax;
ftot(2,1)=ftot(2,1)+dfax;  
%% MOMENTS IN ELASTIC COMPONENT AT BEGINING OF STEP
bmel(1,1)=bmtot(1,1)-bmep(1,1);
bmel(2,1)=bmtot(2,1)-bmep(2,1);
%% LINEAR MOMENT INCREMENTS FOR ELASTO-PLASTIC COMPONENT - SET IN DBM
[dbm] = BMCAO2(dvr,kody,ek11,ek12,ek22,ek22h,ek11h);
%% TRACE NONLINEAR PATH FOR ELASTO-PLASTIC COMPONENT---state determination
facac=0.0;
while (facac<0.999999)
    factor=1.0-facac;
    % PLASTIC HINGE ROTATIONS
    kod=kody(1,1)+kody(2,1)-1.0;
    if(kod>0)
        % hinges at both ends
        dpr(1,1)=dvr(1,1);
        dpr(2,1)=dvr(2,1);
    elseif(kod==0)
        % hinge at one end only
        dpr(1,1)=dvr(1,1)+pr21*dvr(2,1);
        dpr(2,1)=dvr(2,1)+pr12*dvr(1,1);
    else
         %never executed
    end
         
    % CALCULATE WHICH END HAS NEXT EVENT IF YIELDS, SET KFAC=IEND AND BBMY=YIELD VALUE
    % SET EVENT FACTOR IN FACTOR
    kfac=3;
    for iend=1:2
        if (kody(iend,1)==0.0)
            dbmm=dbm(iend,1);
            % elastic, get factor for status change(no hinge at end)
            if (dbmm<0.0)
                dbmo=bmy(iend,2)-bmep(iend,1);
                if(dbmo>=dbmm) 
                    fac=dbmo/dbmm;
                else
                    fac=2.0;
                end 
                if (fac<=factor)
                    factor=fac;
                    bbmy=bmy(iend,2);
                    kfac=iend;
                end
            elseif(dbmm>0.0)
                dbmo=bmy(iend,1)-bmep(iend,1);
                if(dbmo<=dbmm) 
                    fac=dbmo/dbmm;
                else
                    fac=2.0;
                end 
                if (fac<=factor)
                    factor=fac;
                    bbmy=bmy(iend,1);
                    kfac=iend;
                end
            else
            end
        else
            % hinge at this end
            if(bmep(iend,1)*dpr(iend,1)<0.0)
            % unloading (plastic work negative)
                factor=0.0;
                kfac=0.0;
                kody(iend,1)=0.0;
            else
                % continuing to yield (plastic work positive)
            end
        end
    end
    % UPDATE BENDING STATE AND CALCULATE BENDING ENERGY
    % dbm= elastic increment - use if elastic bbmy= yield value - use if yields
    if(kfac~=0)
        for iend=1:2
            if(iend==kfac)
                % new hinge at this end
                bmep(iend,1)=bbmy;
                kody(iend,1)=1;
            elseif(kody(iend,1)==0)
                % this end remains elastic
                dmep=factor*dbm(iend,1);
                bmep(iend,1)=bmep(iend,1)+dmep;
            else
                % this end remains plastic
                dppr=factor*dpr(iend,1);
                prtot(iend,1)=prtot(iend,1)+dppr;
                if (dppr<0.0)
                    pracn(iend,1)=pracn(iend,1)+dppr;
                else
                    pracp(iend,1)=pracp(iend,1)+dppr;
                end
            end
        end
    else
        % unloads - factor=0.
    end
    % CHECK COMPLETION OF CYCLE
    facac=facac+factor;
    if (facac<0.99999)
        % cycle not completed, calculate new moment increments
        [dbm] = BMCAO2(dvr,kody,ek11,ek12,ek22,ek22h,ek11h);
    end
end
%% YIELD MOMENTS FOR NEXT STEP
if(ksurf==1)
    [bmy] = YMOM02(ftot,pmx,a1,a2,bmy);
    % CHECK YIELD SURFACE OVERSHOOT
    for iend=1:2
        if (kody(iend,1)~=0.0)
        % inelastic on old surface
            if (bmep(iend,1)>bmy(iend,1)) 
                % inelastic positive on new surface also
                bmep(iend,1)=bmy(iend,1);
            elseif (bmep(iend,1)<bmy(iend,2))
                % inelastic negative on new surface also
                bmep(iend,1)=bmy(iend,2);
            elseif ((bmep(iend,1)<(bmy(iend,1)*0.98)) && (bmep(iend,1)>(bmy(iend,2)*0.98)))
                % moves inside new surface by > 2% - reset yield code
                kody(iend,1)=0;
            else
            end
        else
            % elastic on old surface
            if (bmep(iend,1)>bmy(iend,1))
                % inelastic positive on new surface
                bmep(iend,1)=bmy(iend,1);
                kody(iend,1)=1;
            elseif (bmep(iend,1)<=bmy(iend,2))
                % inelastic negative on new surface
                bmep(iend,1)=bmy(iend,2);
                kody(iend,1)=1;
            else
            end
        end
    end
end
%% UPDATE TOTAL FORCES
dsf=(bmtot(1,1)+ bmtot(2,1))/fl;
ppsh=psh/(1.0-psh);
dmeli=(ek11*dvr(1,1)+ek12*dvr(2,1))*ppsh+bmel(1,1);
dmelj=(ek12*dvr(1,1)+ ek22*dvr(2,1))*ppsh+bmel(2,1);
bmtot(1,1)=bmep(1,1)+dmeli;
bmtot(2,1)=bmep(2,1)+dmelj;
dsf=dsf-(bmtot(1,1)+bmtot(2,1))/fl;
sftot(1,1)=sftot(1,1)-dsf;
sftot(2,1)=sftot(2,1)+dsf;

RF = ELASO2(ndof,ftot,cosa,sina,sftot,bmtot);





%%%%%%% FUNCTIONS %%%%%%%%%
function [bmy] = YMOM02(ftot,pmx,a1,a2,bmy)
facc=-1.0;
for iend = 1 : 2
    % Change sign of axial force and end 1
    fft = ftot(iend,1) * facc;
    facc = 1;
    fac = 1;
    for j = 1 : 2
        fac = -fac;
        yieldcalc = 0;  % flag if the yield moment is calculated inside 
                        % this next for loop
        for i = 1 : 3
            if (fft < pmx(i,j,iend))
                yieldcalc = 1;  % set flag since the condition was met
                % Calculate yield moment (M = a2 + a1P)
                bbmy = a2(i,j,iend) - a1(i,j,iend) * fft;
                if (fac * bbmy > 0) 
                    % Axial force is beyond Pc and Pt
                    bbmy = 0;
                end
                bmy(iend,j) = bbmy;
            end
        end
        % Only calculate yield moment if it wasn't calculated in the above
        % for loop
        if (yieldcalc == 0)
            i = 4;
            % Calculate yield moment (M = a2 + a1P)
            bbmy = a2(i,j,iend) - a1(i,j,iend) * fft;
            if (fac * bbmy > 0) 
                % Axial force is beyond Pc and Pt
                bbmy = 0;
            end
            bmy(iend,j) = bbmy;
        end
    end
end
%c ---------------------------------INTERCHANGE BMY(1,1) AND BMY(1,2) AND
%c ------------------------------AND ALSO CHANGE SIGN OF MOMENTS AT END 1
fac=-bmy(1,1);
bmy(1,1)=-bmy(1,2);
bmy(1,2)=fac;
      
      
      
      
      
function [dbm] = BMCAO2(dvr,kody,ek11,ek12,ek22,ek22h,ek11h)
dbm=zeros(2,1);
% c ------------------SET KYY TO INDICATE TYPE OF ELEMENT STIFFNESS TO USE
      kyy=kody(1,1)+2*kody(2,1)+1;
      if(kyy==1)
%c---no hinge at either end
        dbm(1,1)=ek11*dvr(1,1)+ek12*dvr(2,1);
        dbm(2,1)=ek12*dvr(1,1)+ek22*dvr(2,1);
      elseif(kyy==2)
%c---hinge at end 1
        dbm(1,1)=0.0;
        dbm(2,1)=ek22h*dvr(2,1);
      elseif(kyy==3)
%c---hinge at end 2
        dbm(1,1)=ek11h*dvr(1,1);
        dbm(2,1)=0.0;
      elseif(kyy==4)
%c---hinges at both end
        dbm(1,1)=0.0;
        dbm(2,1)=0.0;
       else
           %never executed
      end
      
      
      
      
      
      
      
      
      
      
   %%
function [relas] = ELASO2(ndof,ftot,cosa,sina,sftot,bmtot)
%%
relas=zeros(ndof,1);
%BASIC RESISTING FORCES
      relas(1,1)=(ftot(1,1)-0)*cosa-(sftot(1,1)-0)*sina;
      relas(2,1)=(ftot(1,1)-0)*sina+(sftot(1,1)-0)*cosa;
      relas(3,1)=bmtot(1,1)-0-0;
      relas(4,1)=(ftot(2,1)-0)*cosa-(sftot(2,1)-0)*sina;
      relas(5,1)=(ftot(2,1)-0)*sina+(sftot(2,1)-0)*cosa;
      relas(6,1)=bmtot(2,1)-0-0;
%%







%%
function [dvax,dvr] = ELDFO2(ddise,f1,cosa, sina) 
%%
dvr=zeros(2,1);
%DEFORMATION INCREMENTS OR DEFORMATION RATES
      dvax=cosa*(ddise(4,1)-ddise(1,1))+sina*(ddise(5,1)-ddise(2,1));
      rot=(sina*(ddise(4,1)-ddise(1,1))+cosa*(ddise(2,1)-ddise(5,1)))/f1;
      dvr(1,1)=ddise(3,1)+rot;
      dvr(2,1)=ddise(6,1)+rot;
%%

== matlab function Form Total Restoring Force Vector/Form Restoring Force Vector ==
  data: Nodes_muxed input inherited; RF_muxed input inherited; TotalRF output inherited
function TotalRF = eml(Nodes_muxed,RF_muxed)
% This block supports the Embedded MATLAB subset.
% See the help menu for details. 

NumFreeDOF = 12;
TotalRF = zeros(NumFreeDOF,1);

for i = 2:2:length(Nodes_muxed)
    N1 = Nodes_muxed(i-1);
    N2 = Nodes_muxed(i);
    if (3 * N1) <= NumFreeDOF
        TotalRF(N1 * 3 - 2, 1) = RF_muxed(1+(6*(i-2)/2)) + TotalRF(N1 * 3 - 2, 1);
        TotalRF(N1 * 3 - 1, 1) = RF_muxed(2+(6*(i-2)/2)) + TotalRF(N1 * 3 - 1, 1);
        TotalRF(N1 * 3, 1) = RF_muxed(3+(6*(i-2)/2)) + TotalRF(N1 * 3, 1);
    end
    if (3 * N2) <= NumFreeDOF
        TotalRF(N2 * 3 - 2, 1) = RF_muxed(4+(6*(i-2)/2)) + TotalRF(N2 * 3 - 2, 1);
        TotalRF(N2 * 3 - 1, 1) = RF_muxed(5+(6*(i-2)/2)) + TotalRF(N2 * 3 - 1, 1);
        TotalRF(N2 * 3, 1) = RF_muxed(6+(6*(i-2)/2)) + TotalRF(N2 * 3, 1);
    end
end

== matlab function Generate Type 1 Element Restoring Force/Type 1 Element RF ==
  data: Nodes output inherited; Element input inherited; RF output inherited; NumFreeDOF input inherited; Displacement input inherited
% get restoring force for the element
% returns (6x1) restoring force vector of element in global coordinates
function [Nodes,RF] = eml(Element, NumFreeDOF, Displacement)

%% Input mapping
Node1ID = Element(1);
Node1Xcoord = Element(2);
Node1Ycoord = Element(3);
Node2ID = Element(4);
Node2Xcoord = Element(5);
Node2Ycoord = Element(6);
MaterialE = Element(7);
Area = Element(8);
Inertia = Element(9);
Nodes = [Node1ID,Node2ID];

% Get distance between nodes
I1 = Node1ID;
I2 = Node2ID;
X21 = Node2Xcoord - Node1Xcoord;
Y21 = Node2Ycoord - Node1Ycoord;
EL = sqrt(X21 * X21 + Y21 * Y21);
EAL = MaterialE * Area / EL;
EIZL = MaterialE * Inertia / EL;
%calculation of density (the uniform load is only taken into account)
SEP = zeros(6);
SEP(1, 1) = EAL;
SEP(1, 4) = -EAL;
SEP(4, 4) = EAL;
SEP(2, 2) = 12 * EIZL / EL ^ 2;
SEP(2, 3) = 6 * EIZL / EL;
SEP(2, 5) = -SEP(2, 2);
SEP(2, 6) = SEP(2, 3);
SEP(3, 3) = 4 * EIZL;
SEP(3, 5) = -6 * EIZL / EL;
SEP(3, 6) = 2 * EIZL;
SEP(5, 5) = 12 * EIZL / EL ^ 2;
SEP(5, 6) = -6 * EIZL / EL;
SEP(6, 6) = 4 * EIZL;
for i = 1:6
   for j = i:6
      SEP(j, i) = SEP(i, j);
   end
end
DCOS = zeros(3,3);
DCOS(1, 1) = X21 / EL;
DCOS(1, 2) = Y21 / EL;
DCOS(1, 3) = 0;
DCOS(2, 1) = -DCOS(1, 2);
DCOS(2, 2) = DCOS(1, 1);
DCOS(2, 3) = 0;
DCOS(3, 1) = 0;
DCOS(3, 2) = 0;
DCOS(3, 3) = 1;
ALMBDA = zeros(6);       
for i = 1:2
   IK = 3 * (i - 1);
   for j = 1:3
      for k = 1:3
         ALMBDA(j + IK, k + IK) = DCOS(j, k);
      end
   end
end
SE = SEP * ALMBDA;
SEP = SE;
SE = ALMBDA' * SEP;
%create the displacement Ue (6x1) vector of the element in global coordinates
Ue = zeros(6,1);
if (I1 * 3) <= NumFreeDOF
    Ue(1, 1) = Displacement(I1 * 3 - 2, 1);
    Ue(2, 1) = Displacement(I1 * 3 - 1, 1);
    Ue(3, 1) = Displacement(I1 * 3, 1);
end
if (I2 * 3) <= NumFreeDOF
    Ue(4, 1) = Displacement(I2 * 3 - 2, 1);
    Ue(5, 1) = Displacement(I2 * 3 - 1, 1);
    Ue(6, 1) = Displacement(I2 * 3, 1);
end
RF = SE * Ue;  %resisting (6x1) resisting force vector of element in global coordinates

== matlab function Generate Type 2 Element Restoring Force/Type 2 Element RF ==
  data: Nodes output inherited; Element input inherited; RF output inherited; NumFreeDOF input inherited; Displacement input inherited
% get restoring force for the element
% returns (6x1) restoring force vector of element in global coordinates
function [Nodes,RF] = fcn(Element, NumFreeDOF, Displacement)

%% Input mapping
Node1ID = Element(1);
Node2ID = Element(2);
Stiffness = Element(3);
Nodes = [Node1ID,Node2ID];

% Get distance between nodes
I1 = Node1ID;
I2 = Node2ID;

% preset arrays
SE = zeros(6,6);
    
SE(1, 1) = Stiffness;
SE(1, 4) = -Stiffness;
SE(4, 4) = Stiffness;
SE(4, 1) = SE(1,4);
%create the displacement Ue (6x1) vector of the element in global coordinates
Ue = zeros(6, 1);
if (I1 * 3) <= NumFreeDOF
    Ue(1, 1) = Displacement(I1 * 3 - 2, 1);
    Ue(2, 1) = Displacement(I1 * 3 - 1, 1);
    Ue(3, 1) = Displacement(I1 * 3, 1);
end
if (I2 * 3) <= NumFreeDOF
    Ue(4, 1) = Displacement(I2 * 3 - 2, 1);
    Ue(5, 1) = Displacement(I2 * 3 - 1, 1);
    Ue(6, 1) = Displacement(I2 * 3, 1);
end
RF = SE*Ue;  %resisting (6x1) resisting force vector of element in global coordinates

== matlab function Generate Acceleration Vector/Generate Acceleration Vector ==
  data: TotalRF input inherited; PEFF input inherited; M_FreeInv input inherited; Acceleration output inherited; C_Free input inherited; Velocity input inherited; step_count input inherited
function Acceleration = eml(TotalRF,PEFF,M_FreeInv,C_Free,Velocity,step_count)
% This block supports the Embedded MATLAB subset.
% See the help menu for details. 

Acceleration = M_FreeInv * (PEFF(step_count,:)' - C_Free * Velocity - TotalRF);

== matlab function Generate Command Vectors/Generate Command Vectors ==
  data: Timestep input inherited; Displacement_v output inherited; Beta1 input inherited; Beta2 input inherited; Displacement input inherited; Velocity input inherited; Acceleration input inherited; Velocity_v output inherited
function [Displacement_v,Velocity_v] = eml(Timestep, Beta1, Beta2, Displacement, Velocity, Acceleration)
% This block supports the Embedded MATLAB subset.
% See the help menu for details. 

Displacement_v = Displacement + Timestep*Velocity + Beta2*Timestep^2*Acceleration;
Velocity_v = Velocity + Beta1*Timestep*Acceleration;
